simulink model "WS22"  (R2025b)
settings: Solver=ode45  StartTime=0.0  StopTime=30.0  RelTol=1e-3
values from neighbouring files (symbols this model uses):
  Beq = 4.3    [WS2.m]
  Bp = 0.0024    [WS2.m]
  g = 9.81    [WS2.m]
  Ip = 0.0079    [WS2.m]
  lp = 0.3302    [WS2.m]
  Mc = 0.7031    [WS2.m]
  Mp = 0.23    [WS2.m]

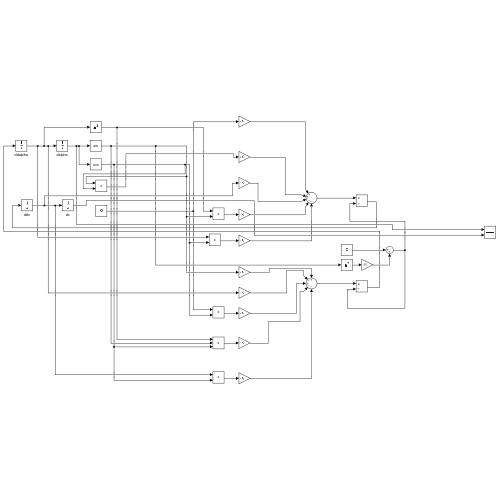
[thumbnail: Simulink's stored preview of the top-level diagram]
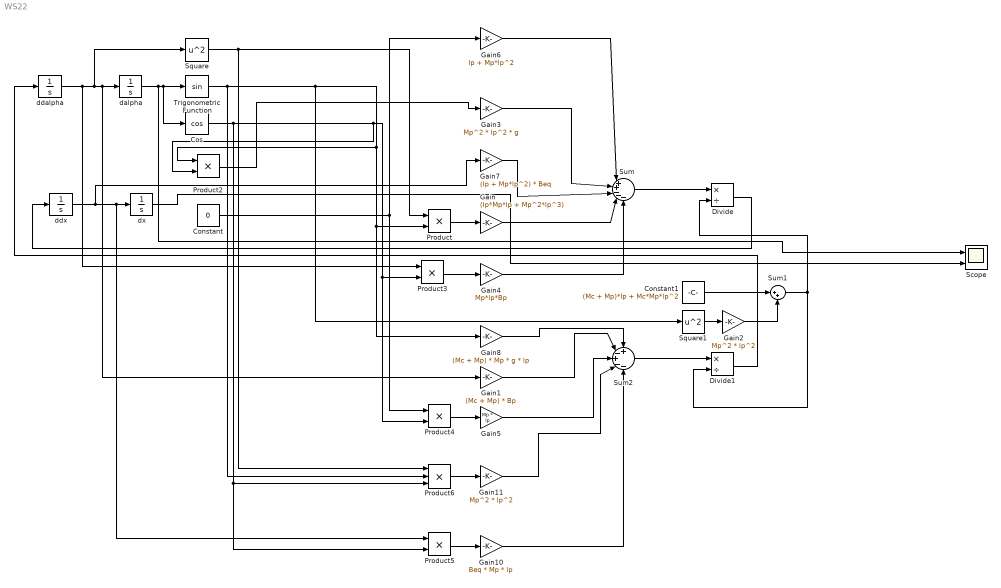
== system WS22 ==
  Constant : Constant  Value=0
  Constant1 : Constant  Value=(Mc + Mp)*Ip + Mc*Mp*lp^2
  Cos : Trigonometry  Operator=cos
  Divide : Product  Inputs=*/
  Divide1 : Product  Inputs=*/
  Gain : Gain  Gain=(Ip*Mp*lp + Mp^2*lp^3)
  Gain1 : Gain  Gain=(Mc + Mp) * Bp
  Gain10 : Gain  Gain=Beq * Mp * lp
  Gain11 : Gain  Gain=Mp^2 * lp^2
  Gain2 : Gain  Gain=Mp^2 * lp^2
  Gain3 : Gain  Gain=Mp^2 * lp^2 * g
  Gain4 : Gain  Gain=Mp*lp*Bp
  Gain5 : Gain  Gain=Mp * lp
  Gain6 : Gain  Gain=Ip + Mp*lp^2
  Gain7 : Gain  Gain=(Ip + Mp*lp^2) * Beq
  Gain8 : Gain  Gain=(Mc + Mp) * Mp * g * lp
  Product{,2..5} (5 alike) : Product
  Product6 : Product  Inputs=3
  Scope : Scope  NumInputPorts=2
      settings: ActiveDisplayYMinimum=-7.9868900411222956  ActiveDisplayYMaximum=16.767543246003989
  Square : Math  Operator=square
  Square1 : Math  Operator=square
  Sum : Sum  Inputs=|++---
  Sum1 : Sum  Inputs=|++
  Sum2 : Sum  Inputs=+-+--
  Trigonometric Function : Trigonometry
  dalpha : Integrator  InitialCondition=1*pi/180
  ddalpha : Integrator
  ddx : Integrator
  dx : Integrator
  wires:
  ddx/1 -> Gain7/1, Product5/1, dx/1
  ddalpha/1 -> Product3/1, Square/1, Gain1/1, dalpha/1
  dalpha/1 -> Scope/1, Cos/1, Trigonometric Function/1
  Gain6/1 -> Sum/1
  Trigonometric Function/1 -> Square1/1, Product/2, Gain8/1, Product2/1, Product6/2
  Cos/1 -> Product5/2, Product6/3, Product4/2, Product3/2, Product2/2
  Product2/1 -> Gain3/1
  Gain3/1 -> Sum/2
  Gain7/1 -> Sum/3
  Square/1 -> Product6/1, Product/1
  Product/1 -> Gain/1
  Gain/1 -> Sum/4
  Product3/1 -> Gain4/1
  Gain4/1 -> Sum/5
  Sum/1 -> Divide/1
  Gain8/1 -> Sum2/1
  Gain1/1 -> Sum2/2
  Constant/1 -> Product4/1, Gain6/1
  Product4/1 -> Gain5/1
  Gain5/1 -> Sum2/3
  Product6/1 -> Gain11/1
  Gain11/1 -> Sum2/4
  Product5/1 -> Gain10/1
  Gain10/1 -> Sum2/5
  Sum2/1 -> Divide1/1
  Constant1/1 -> Sum1/1
  Square1/1 -> Gain2/1
  Gain2/1 -> Sum1/2
  Sum1/1 -> Divide1/2, Divide/2
  Divide/1 -> ddx/1
  Divide1/1 -> ddalpha/1
  dx/1 -> Scope/2
